simulink model "lab3"  (R2024a)
settings: Solver=VariableStepAuto  StartTime=0.0  StopTime=10.0  MaxStep=1/128  RelTol=1e-3
settings Model: Creator=gm54508  LastModifiedBy=gm54508

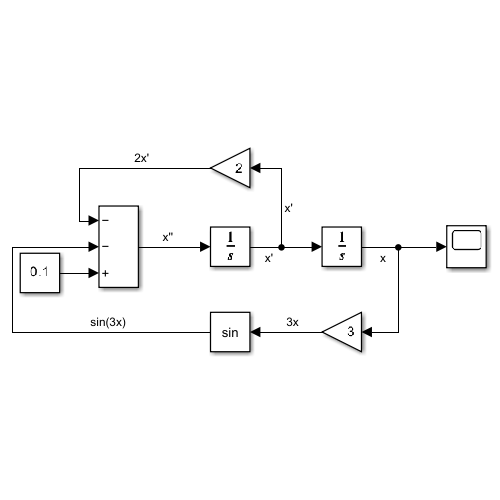
[thumbnail: Simulink's stored preview of the top-level diagram]
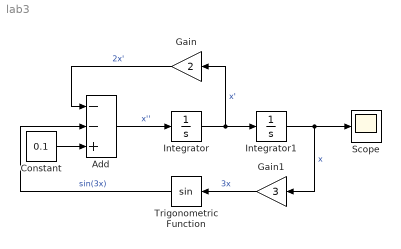
== system lab3 ==
  Add : Sum  Inputs=--+
  Constant : Constant  Value=0.1
  Gain : Gain  Gain=2
  Gain1 : Gain  Gain=3
  Integrator : Integrator  InitialCondition=2
  Integrator1 : Integrator
  Scope : Scope
  Trigonometric Function : Trigonometry
  wires:
  Integrator/1 -> Gain/1, Integrator1/1  "x'"
  Add/1 -> Integrator/1  "x''"
  Integrator1/1 -> Gain1/1, Scope/1  "x"
  Constant/1 -> Add/3
  Gain/1 -> Add/1  "2x'"
  Gain1/1 -> Trigonometric Function/1  "3x"
  Trigonometric Function/1 -> Add/2  "sin(3x)"
